simulink model "TST_CoTS_MechDem"  (R2016b)
settings: Solver=FixedStepDiscrete  StartTime=0.0  StopTime=simTime  FixedStep=sampleTime  RelTol=1e-3
values from neighbouring files (symbols this model uses):
  testCase = 1    [initTST_CoTS_MechDem_001.m]
libraries: simulink x6, UnitTest_Lib x4
settings Model: Creator=xinchangran  LastModifiedBy=xinchangran
settings DebuggingCC: SignalRangeChecking=error

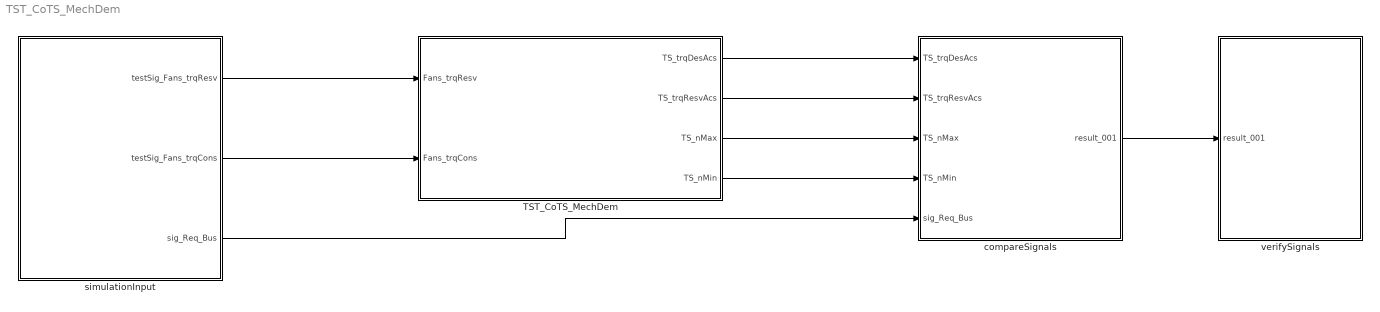
== system TST_CoTS_MechDem ==
  TST_CoTS_MechDem : Subsystem
  compareSignals : Subsystem
  simulationInput : Subsystem
  verifySignals : Subsystem
  wires:
  simulationInput/1(testSig_Fans_trqResv) -> TST_CoTS_MechDem/1(Fans_trqResv)
  simulationInput/2(testSig_Fans_trqCons) -> TST_CoTS_MechDem/2(Fans_trqCons)
  TST_CoTS_MechDem/1(TS_trqDesAcs) -> compareSignals/1(TS_trqDesAcs)
  TST_CoTS_MechDem/2(TS_trqResvAcs) -> compareSignals/2(TS_trqResvAcs)
  TST_CoTS_MechDem/3(TS_nMax) -> compareSignals/3(TS_nMax)
  TST_CoTS_MechDem/4(TS_nMin) -> compareSignals/4(TS_nMin)
  simulationInput/3(sig_Req_Bus) -> compareSignals/5(sig_Req_Bus)
  compareSignals/1(result_001) -> verifySignals/1(result_001)

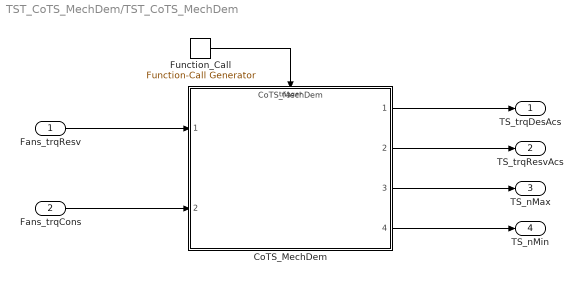
== system TST_CoTS_MechDem/TST_CoTS_MechDem ==
  Fans_trqResv : Inport
  Fans_trqCons : Inport  Port=2
  CoTS_MechDem : ModelReference  ModelNameDialog=CoTS_MechDem  SimulationMode=Normal  ModelReferenceVersion=1.18  TriggerPortName=function  TriggerPortTriggerType=function-call  TriggerPortStatesWhenEnabling=held
  Function_Call : simulink/Ports & Subsystems/Function-Call Generator  sample_time=sampleTime  numberOfIterations=1
  TS_trqDesAcs : Outport
  TS_trqResvAcs : Outport  Port=2
  TS_nMax : Outport  Port=3
  TS_nMin : Outport  Port=4
  wires:
  Function_Call/1 -> CoTS_MechDem/Trigger
  Fans_trqResv/1 -> CoTS_MechDem/1
  Fans_trqCons/1 -> CoTS_MechDem/2
  CoTS_MechDem/1 -> TS_trqDesAcs/1
  CoTS_MechDem/2 -> TS_trqResvAcs/1
  CoTS_MechDem/3 -> TS_nMax/1
  CoTS_MechDem/4 -> TS_nMin/1

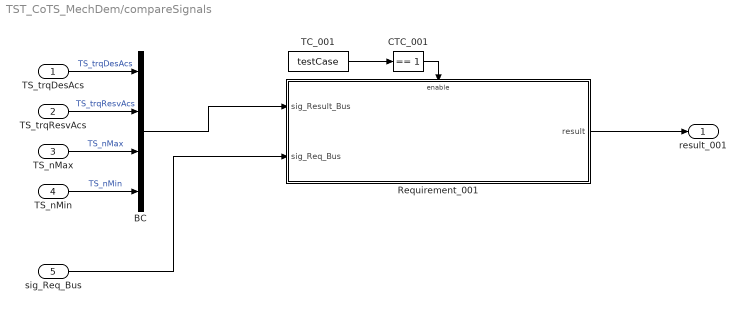
== system TST_CoTS_MechDem/compareSignals ==
  TS_trqDesAcs : Inport
  TS_trqResvAcs : Inport  Port=2
  TS_nMax : Inport  Port=3
  TS_nMin : Inport  Port=4
  sig_Req_Bus : Inport  Port=5
  BC : BusCreator  Inputs=4
  CTC_001 : simulink/Logic and Bit Operations/Compare To Constant  relop===  const=1  OutDataTypeStr=boolean
  Requirement_001 : Subsystem
  TC_001 : Constant  Value=testCase
  result_001 : Outport
  wires:
  TS_trqDesAcs/1 -> BC/1  "TS_trqDesAcs"
  TS_trqResvAcs/1 -> BC/2  "TS_trqResvAcs"
  TS_nMax/1 -> BC/3  "TS_nMax"
  TS_nMin/1 -> BC/4  "TS_nMin"
  TC_001/1 -> CTC_001/1
  CTC_001/1 -> Requirement_001/Enable
  sig_Req_Bus/1 -> Requirement_001/2(sig_Req_Bus)
  BC/1 -> Requirement_001/1(sig_Result_Bus)
  Requirement_001/1(result) -> result_001/1

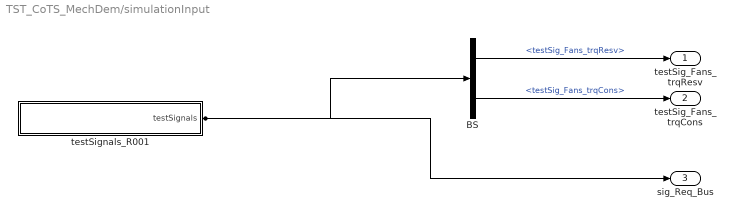
== system TST_CoTS_MechDem/simulationInput ==
  BS : BusSelector  OutputSignals=testSig_Fans_trqResv,testSig_Fans_trqCons
  testSignals_R001 : Subsystem
  testSig_Fans_trqResv : Outport
  testSig_Fans_trqCons : Outport  Port=2
  sig_Req_Bus : Outport  Port=3
  wires:
  BS/1 -> testSig_Fans_trqResv/1  "<testSig_Fans_trqResv>"
  BS/2 -> testSig_Fans_trqCons/1  "<testSig_Fans_trqCons>"
  testSignals_R001/1(testSignals) -> BS/1, sig_Req_Bus/1

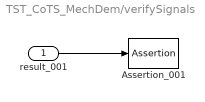
== system TST_CoTS_MechDem/verifySignals ==
  result_001 : Inport
  Assertion_001 : Assertion  Enabled=off
  wires:
  result_001/1 -> Assertion_001/1

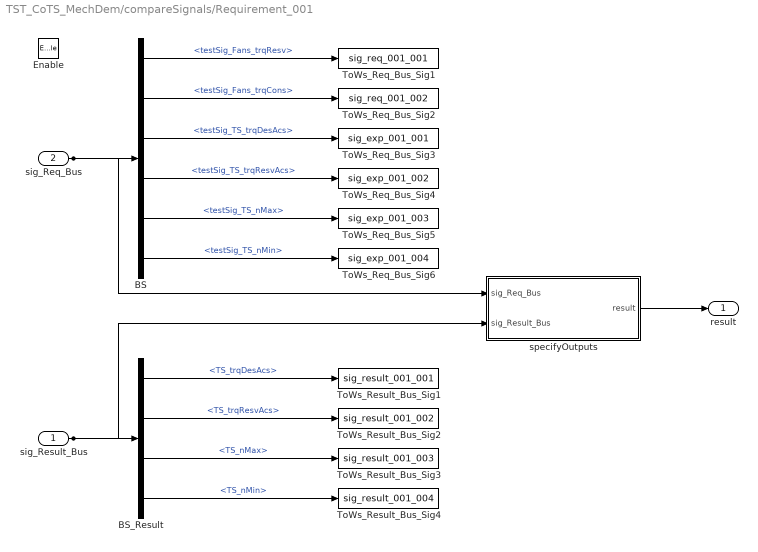
== system TST_CoTS_MechDem/compareSignals/Requirement_001 ==
  sig_Result_Bus : Inport
  sig_Req_Bus : Inport  Port=2
  Enable : EnablePort
  BS : BusSelector  OutputSignals=testSig_Fans_trqResv,testSig_Fans_trqCons,testSig_TS_trqDesAcs,testSig_TS_trqResvAcs,testSig_TS_nMax,testSig_TS_nMin
  BS_Result : BusSelector  OutputSignals=TS_trqDesAcs,TS_trqResvAcs,TS_nMax,TS_nMin
  ToWs_Req_Bus_Sig1 : ToWorkspace  VariableName=sig_req_001_001  SaveFormat=Structure With Time
  ToWs_Req_Bus_Sig2 : ToWorkspace  VariableName=sig_req_001_002  SaveFormat=Structure With Time
  ToWs_Req_Bus_Sig3 : ToWorkspace  VariableName=sig_exp_001_001  SaveFormat=Structure With Time
  ToWs_Req_Bus_Sig4 : ToWorkspace  VariableName=sig_exp_001_002  SaveFormat=Structure With Time
  ToWs_Req_Bus_Sig5 : ToWorkspace  VariableName=sig_exp_001_003  SaveFormat=Structure With Time
  ToWs_Req_Bus_Sig6 : ToWorkspace  VariableName=sig_exp_001_004  SaveFormat=Structure With Time
  ToWs_Result_Bus_Sig1 : ToWorkspace  VariableName=sig_result_001_001  SaveFormat=Structure With Time
  ToWs_Result_Bus_Sig2 : ToWorkspace  VariableName=sig_result_001_002  SaveFormat=Structure With Time
  ToWs_Result_Bus_Sig3 : ToWorkspace  VariableName=sig_result_001_003  SaveFormat=Structure With Time
  ToWs_Result_Bus_Sig4 : ToWorkspace  VariableName=sig_result_001_004  SaveFormat=Structure With Time
  specifyOutputs : Subsystem
  result : Outport
  wires:
  sig_Req_Bus/1 -> BS/1, specifyOutputs/1(sig_Req_Bus)
  BS/1 -> ToWs_Req_Bus_Sig1/1  "<testSig_Fans_trqResv>"
  BS/2 -> ToWs_Req_Bus_Sig2/1  "<testSig_Fans_trqCons>"
  BS/3 -> ToWs_Req_Bus_Sig3/1  "<testSig_TS_trqDesAcs>"
  BS/4 -> ToWs_Req_Bus_Sig4/1  "<testSig_TS_trqResvAcs>"
  BS/5 -> ToWs_Req_Bus_Sig5/1  "<testSig_TS_nMax>"
  BS/6 -> ToWs_Req_Bus_Sig6/1  "<testSig_TS_nMin>"
  sig_Result_Bus/1 -> BS_Result/1, specifyOutputs/2(sig_Result_Bus)
  BS_Result/1 -> ToWs_Result_Bus_Sig1/1  "<TS_trqDesAcs>"
  BS_Result/2 -> ToWs_Result_Bus_Sig2/1  "<TS_trqResvAcs>"
  BS_Result/3 -> ToWs_Result_Bus_Sig3/1  "<TS_nMax>"
  BS_Result/4 -> ToWs_Result_Bus_Sig4/1  "<TS_nMin>"
  specifyOutputs/1(result) -> result/1

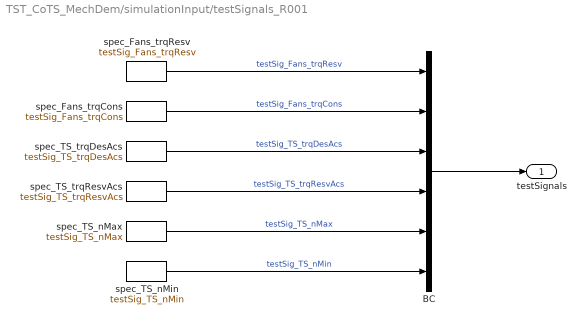
== system TST_CoTS_MechDem/simulationInput/testSignals_R001 ==
  BC : BusCreator  Inputs=6
  spec_Fans_trqCons : FromWorkspace  VariableName=testSig_Fans_trqCons  Interpolate=off  OutputAfterFinalValue=Holding final value
  spec_Fans_trqResv : FromWorkspace  VariableName=testSig_Fans_trqResv  Interpolate=off  OutputAfterFinalValue=Holding final value
  spec_TS_nMax : FromWorkspace  VariableName=testSig_TS_nMax  Interpolate=off  OutputAfterFinalValue=Holding final value
  spec_TS_nMin : FromWorkspace  VariableName=testSig_TS_nMin  Interpolate=off  OutputAfterFinalValue=Holding final value
  spec_TS_trqDesAcs : FromWorkspace  VariableName=testSig_TS_trqDesAcs  Interpolate=off  OutputAfterFinalValue=Holding final value
  spec_TS_trqResvAcs : FromWorkspace  VariableName=testSig_TS_trqResvAcs  Interpolate=off  OutputAfterFinalValue=Holding final value
  testSignals : Outport
  wires:
  BC/1 -> testSignals/1
  spec_Fans_trqResv/1 -> BC/1  "testSig_Fans_trqResv"
  spec_Fans_trqCons/1 -> BC/2  "testSig_Fans_trqCons"
  spec_TS_trqDesAcs/1 -> BC/3  "testSig_TS_trqDesAcs"
  spec_TS_trqResvAcs/1 -> BC/4  "testSig_TS_trqResvAcs"
  spec_TS_nMax/1 -> BC/5  "testSig_TS_nMax"
  spec_TS_nMin/1 -> BC/6  "testSig_TS_nMin"

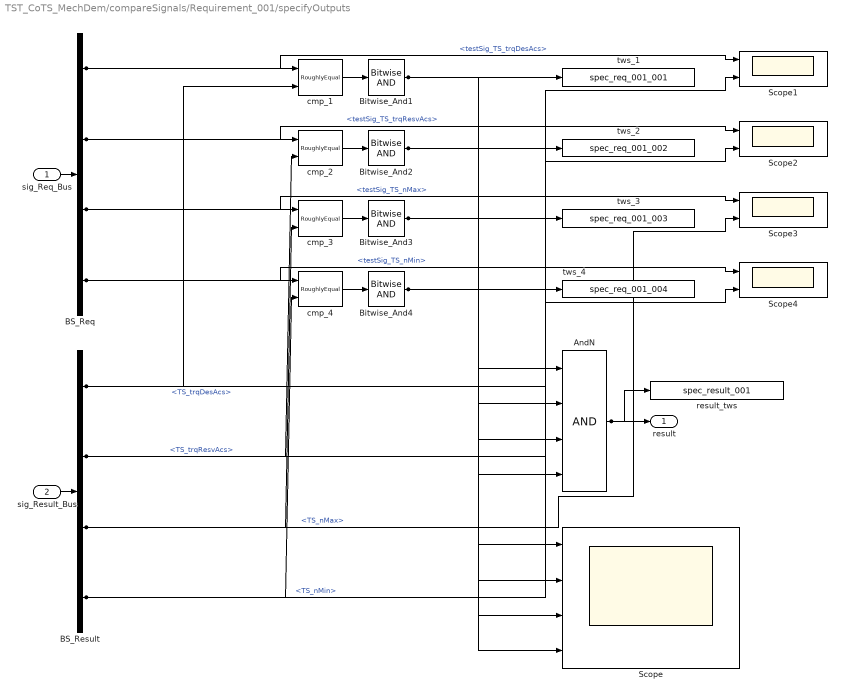
== system TST_CoTS_MechDem/compareSignals/Requirement_001/specifyOutputs ==
  sig_Req_Bus : Inport
  sig_Result_Bus : Inport  Port=2
  AndN : Logic  Inputs=4
  BS_Req : BusSelector  OutputSignals=testSig_TS_trqDesAcs,testSig_TS_trqResvAcs,testSig_TS_nMax,testSig_TS_nMin
  BS_Result : BusSelector  OutputSignals=TS_trqDesAcs,TS_trqResvAcs,TS_nMax,TS_nMin
  Bitwise_And{1..4} (4 alike) : simulink/Logic and Bit Operations/Bitwise Operator  logicop=AND  UseBitMask=off  BitMask=bin2dec('11011001')  BitMaskRealWorld=Stored Integer
  Scope : Scope  NumInputPorts=4
  Scope{1..4} (4 alike) : Scope  NumInputPorts=2
  cmp_{1..4} (4 alike) : UnitTest_Lib/RoughlyEqual  slope=0.1
  result_tws : ToWorkspace  VariableName=spec_result_001
  tws_1 : ToWorkspace  VariableName=spec_req_001_001
  tws_2 : ToWorkspace  VariableName=spec_req_001_002
  tws_3 : ToWorkspace  VariableName=spec_req_001_003
  tws_4 : ToWorkspace  VariableName=spec_req_001_004
  result : Outport
  wires:
  sig_Req_Bus/1 -> BS_Req/1
  sig_Result_Bus/1 -> BS_Result/1
  AndN/1 -> result/1, result_tws/1
  BS_Req/1 -> cmp_1/1, Scope1/1  "<testSig_TS_trqDesAcs>"
  BS_Result/1 -> cmp_1/2, Scope1/2  "<TS_trqDesAcs>"
  cmp_1/1 -> Bitwise_And1/1
  Bitwise_And1/1 -> tws_1/1, AndN/1, Scope/1
  BS_Req/2 -> cmp_2/1, Scope2/1  "<testSig_TS_trqResvAcs>"
  BS_Result/2 -> cmp_2/2, Scope2/2  "<TS_trqResvAcs>"
  cmp_2/1 -> Bitwise_And2/1
  Bitwise_And2/1 -> tws_2/1, AndN/2, Scope/2
  BS_Req/3 -> cmp_3/1, Scope3/1  "<testSig_TS_nMax>"
  BS_Result/3 -> cmp_3/2, Scope3/2  "<TS_nMax>"
  cmp_3/1 -> Bitwise_And3/1
  Bitwise_And3/1 -> tws_3/1, AndN/3, Scope/3
  BS_Req/4 -> cmp_4/1, Scope4/1  "<testSig_TS_nMin>"
  BS_Result/4 -> cmp_4/2, Scope4/2  "<TS_nMin>"
  cmp_4/1 -> Bitwise_And4/1
  Bitwise_And4/1 -> tws_4/1, AndN/4, Scope/4
